simulink model "abc"  (R2016a)
settings: Solver=VariableStepAuto  StartTime=0.0  StopTime=end_time  RelTol=1e-3
values from neighbouring files (symbols this model uses):
  Lambdad = 1e-5    (= 1e-05)    [myModel_param.m]
  Lambdaq = 1e-5    (= 1e-05)    [myModel_param.m]
  Li = 0.16e-3    (= 0.00016)    [Model.m]    (also in myModel_param.m)
  ri = 0.1    [Model.m]    (also in myModel_param.m)
  s_1 = [0;0;0]    [myModel_param.m]
  s_2 = [1;0;0]    [myModel_param.m]
  s_3 = [1;1;0]    [myModel_param.m]
  s_4 = [0;1;0]    [myModel_param.m]
  s_5 = [0;1;1]    [myModel_param.m]
  s_6 = [0;0;1]    [myModel_param.m]
  s_7 = [1;0;1]    [myModel_param.m]
  s_8 = [1;1;1]    [myModel_param.m]
  Ts = 1e-4    (= 0.0001)    [Model.m]    (also in myModel_param.m = 0.001)
  wg = 61.25    [Model.m]    (also in myModel_param.m)
undefined symbols (not defined in the file or in its folder): Lambda1, Lambda2, LambdaP, P_ref
libraries: powerlib x12
settings Model: Creator=syf  LastModifiedBy=syf

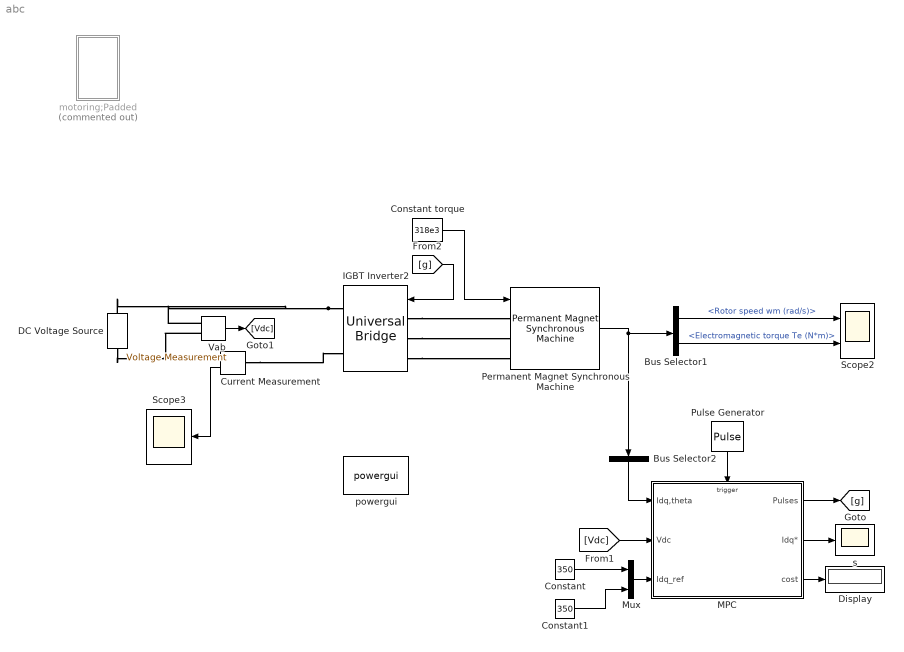
== system abc ==
  Bus Selector1 : BusSelector  OutputSignals=Rotor speed wm (rad/s),Electromagnetic torque Te (N*m)
  Bus Selector2 : BusSelector  OutputSignals=Stator current is_d (A),Stator current is_q (A),Rotor angle thetam (rad)  OutputAsBus=on
  Constant : Constant  Value=350
  Constant torque : Constant  Value=318e3
  Constant1 : Constant  Value=350
  Current Measurement : powerlib/Measurements/Current Measurement  PhasorSimulation=off  OutputType=Complex  PSBequivalent=0
  DC Voltage Source : powerlib/Electrical Sources/DC Voltage Source  Amplitude=540  Measurements=None
  Display : Display
  IGBT Inverter2 : powerlib/Power Electronics/Universal Bridge  Arms=3  SnubberResistance=1e6  SnubberCapacitance=1e-9  Device=IGBT / Diodes  Ron=1e-3  Lon=0  ForwardVoltages="[  0.8  0.8  ]"  ForwardVoltage=.8  GTOparameters=[ 1e-6 , 1e-6 ]  IGBTparameters=[ 1e-6 , 2e-6 ]  Measurements=All voltages and currents  Measurements_2=None  converterType=Rectifier
  MPC : Subsystem  TreatAsAtomicUnit=on
  Mux : Mux  Inputs=2
  Permanent Magnet Synchronous Machine : powerlib/Machines/Permanent Magnet Synchronous Machine  NbPhases=3  FluxDistribution=Sinusoidal  RotorType=Salient-pole  MechanicalLoad=Torque Tm  PresetModel=No  ShowDetailedParameters=on  MeasurementBus=off  Resistance=8.02e-3  Inductance=8.5e-3  dqInductances=[8.5e-3,8.5e-3]  La=2.07e-3  MachineConstant=Flux linkage established by magnets (V.s)  Flux=9.13  VoltageCst=43055.9693  TorqueCst=356.07  Flat=120  Mechanical=[1307e3 0.0004924 26 0]  PolePairs=4  InitialConditions=[0,0, 0,0]  InitialConditions5ph=[0 0 0 0 0 0]  TsPowergui=0  TsBlock=-1  RefAngle=Aligned with phase A axis (original Park)
  Pulse Generator : DiscretePulseGenerator  PulseType=Time based  Period=Ts*0.01  PulseWidth=20
  Scope2 : Scope  NumInputPorts=2
  Scope3 : Scope
  Vab : powerlib/Measurements/Voltage Measurement  Tag=PoWeRsYsTeMmEaSuReMeNt  PhasorSimulation=off  OutputType=Magnitude  PSBequivalent=0
  motoring;Padded : Subsystem  Commented=on
  powergui : powerlib/powergui  Priority=1  SimulationMode=Continuous  SolverType=Tustin/Backward Euler (TBE)  SampleTime=50e-6  frequency=60  SPID=on  DisableSnubberDevices=on  DisableRonSwitches=on  DisableVfSwitches=on  SwTol=0  DisplayEquations=off  Interpol=off  ExternalGateDelay=off  methode=off  Ts=10  FunctionMessages=off  echomessages=off  HookPort=off  EnableUseOfTLC=off  x0status=blocks  frequencyindice=0  Pbase=100e6  ErrMax=1e-4  Iterations=50  UnitsV=kV  UnitsW=MW  buscounter=0  RestoreLinks=warning  ResistiveCurrentMeasurement=off  Frange=[0:2:500]  Ylog=off  Xlog=on  ShowGrid=off  save=off  variable=ZData  structure=0  ZoomFFT=off  StartTime=0.0  cycles=1  DisplayStyle=1  fundamental=60  FreqAxis=off  MaxFrequency=1000  frequencyindicesteady=1  RmsSteady=1  display=off
  s : Scope
  wires:
  Bus Selector1/2 -> Scope2/2  "<Electromagnetic torque Te (N*m)>"
  Bus Selector1/1 -> Scope2/1  "<Rotor speed wm (rad/s)>"
  Pulse Generator/1 -> MPC/Trigger
  Permanent Magnet Synchronous Machine/1 -> Bus Selector2/1, Bus Selector1/1
  [Vdc] -> MPC/2(Vdc)
  MPC/1(Pulses) -> [g]
  Bus Selector2/1 -> MPC/1(Idq,theta)
  Constant torque/1 -> Permanent Magnet Synchronous Machine/1
  Vab/1 -> [Vdc]
  Current Measurement/1 -> Scope3/1
  MPC/2(Idq*) -> s/1
  MPC/3(cost) -> Display/1
  Mux/1 -> MPC/3(Idq_ref)
  Constant/1 -> Mux/1
  Constant1/1 -> Mux/2
  [g] -> IGBT Inverter2/1
  connections:
  Vab/LConn2 -- DC Voltage Source/LConn1 -- Current Measurement/RConn1
  IGBT Inverter2/RConn1 -- Vab/LConn1 -- DC Voltage Source/RConn1
  IGBT Inverter2/LConn3 -- Permanent Magnet Synchronous Machine/LConn3
  Current Measurement/LConn1 -- IGBT Inverter2/RConn2
  IGBT Inverter2/LConn2 -- Permanent Magnet Synchronous Machine/LConn2
  IGBT Inverter2/LConn1 -- Permanent Magnet Synchronous Machine/LConn1

== system abc/MPC ==
  Idq,theta : Inport
  Vdc : Inport  Port=2
  Idq_ref : Inport  Port=3
  Trigger : TriggerPort  VariantControl=Variant
  For Loop : Subsystem  TreatAsAtomicUnit=on
  Gate Pulse Translation for min sw : Subsystem
  Pulses : Outport
  Idq* : Outport  Port=2
  cost : Outport  Port=3
  wires:
  Idq,theta/1 -> For Loop/1(Idq,theta)
  Vdc/1 -> For Loop/2(Vdc)
  Gate Pulse Translation for min sw/1(pulses) -> Pulses/1
  For Loop/1(opti) -> Gate Pulse Translation for min sw/1(i)
  Idq_ref/1 -> For Loop/3(Idq_ref)
  For Loop/2(Idq*) -> Idq*/1
  For Loop/3(cost) -> cost/1

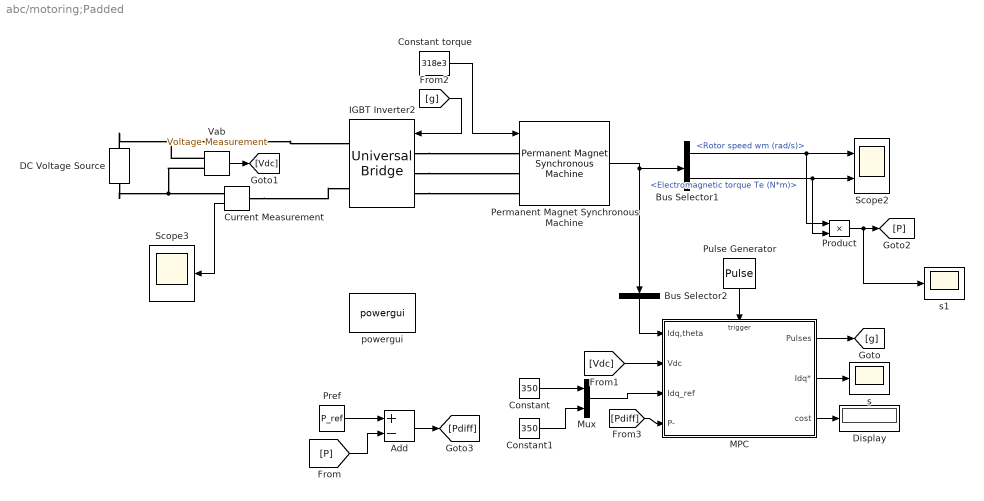
== system abc/motoring;Padded ==
  Add : Sum  Inputs=+-
  Bus Selector1 : BusSelector  OutputSignals=Rotor speed wm (rad/s),Electromagnetic torque Te (N*m)
  Bus Selector2 : BusSelector  OutputSignals=Stator current is_d (A),Stator current is_q (A),Rotor angle thetam (rad)  OutputAsBus=on
  Constant : Constant  Value=350
  Constant torque : Constant  Value=318e3
  Constant1 : Constant  Value=350
  Current Measurement : powerlib/Measurements/Current Measurement  PhasorSimulation=off  OutputType=Complex  PSBequivalent=0
  DC Voltage Source : powerlib/Electrical Sources/DC Voltage Source  Amplitude=540  Measurements=None
  Display : Display
  IGBT Inverter2 : powerlib/Power Electronics/Universal Bridge  Arms=3  SnubberResistance=1e6  SnubberCapacitance=1e-9  Device=IGBT / Diodes  Ron=1e-3  Lon=0  ForwardVoltages="[  0.8  0.8  ]"  ForwardVoltage=.8  GTOparameters=[ 1e-6 , 1e-6 ]  IGBTparameters=[ 1e-6 , 2e-6 ]  Measurements=All voltages and currents  Measurements_2=None  converterType=Rectifier
  MPC : Subsystem  TreatAsAtomicUnit=on
  Mux : Mux  Inputs=2
  Permanent Magnet Synchronous Machine : powerlib/Machines/Permanent Magnet Synchronous Machine  NbPhases=3  FluxDistribution=Sinusoidal  RotorType=Salient-pole  MechanicalLoad=Torque Tm  PresetModel=No  ShowDetailedParameters=on  MeasurementBus=off  Resistance=8.02e-3  Inductance=8.5e-3  dqInductances=[8.5e-3,8.5e-3]  La=2.07e-3  MachineConstant=Flux linkage established by magnets (V.s)  Flux=9.13  VoltageCst=43055.9693  TorqueCst=356.07  Flat=120  Mechanical=[1307e3 0.0004924 26 0]  PolePairs=4  InitialConditions=[0,0, 0,0]  InitialConditions5ph=[0 0 0 0 0 0]  TsPowergui=0  TsBlock=-1  RefAngle=Aligned with phase A axis (original Park)
  Pref : Constant  Value=P_ref
  Product : Product
  Pulse Generator : DiscretePulseGenerator  PulseType=Time based  Period=Ts*0.01  PulseWidth=20
  Scope2 : Scope  NumInputPorts=2
  Scope3 : Scope
  Vab : powerlib/Measurements/Voltage Measurement  Tag=PoWeRsYsTeMmEaSuReMeNt  PhasorSimulation=off  OutputType=Magnitude  PSBequivalent=0
  powergui : powerlib/powergui  Priority=1  SimulationMode=Continuous  SolverType=Tustin/Backward Euler (TBE)  SampleTime=50e-6  frequency=60  SPID=on  DisableSnubberDevices=on  DisableRonSwitches=on  DisableVfSwitches=on  SwTol=0  DisplayEquations=off  Interpol=off  ExternalGateDelay=off  methode=off  Ts=10  FunctionMessages=off  echomessages=off  HookPort=off  EnableUseOfTLC=off  x0status=blocks  frequencyindice=0  Pbase=100e6  ErrMax=1e-4  Iterations=50  UnitsV=kV  UnitsW=MW  buscounter=0  RestoreLinks=warning  ResistiveCurrentMeasurement=off  Frange=[0:2:500]  Ylog=off  Xlog=on  ShowGrid=off  save=off  variable=ZData  structure=0  ZoomFFT=off  StartTime=0.0  cycles=1  DisplayStyle=1  fundamental=60  FreqAxis=off  MaxFrequency=1000  frequencyindicesteady=1  RmsSteady=1  display=off
  s : Scope
  s1 : Scope
  wires:
  [g] -> IGBT Inverter2/1
  Constant1/1 -> Mux/2
  Constant/1 -> Mux/1
  Mux/1 -> MPC/3(Idq_ref)
  MPC/3(cost) -> Display/1
  MPC/2(Idq*) -> s/1
  Current Measurement/1 -> Scope3/1
  Vab/1 -> [Vdc]
  Constant torque/1 -> Permanent Magnet Synchronous Machine/1
  Bus Selector2/1 -> MPC/1(Idq,theta)
  MPC/1(Pulses) -> [g]
  [Vdc] -> MPC/2(Vdc)
  Permanent Magnet Synchronous Machine/1 -> Bus Selector1/1, Bus Selector2/1
  Pulse Generator/1 -> MPC/Trigger
  Bus Selector1/1 -> Product/1, Scope2/1  "<Rotor speed wm (rad/s)>"
  Bus Selector1/2 -> Product/2, Scope2/2  "<Electromagnetic torque Te (N*m)>"
  Product/1 -> s1/1, [P]
  Pref/1 -> Add/1
  [P] -> Add/2
  Add/1 -> [Pdiff]
  [Pdiff] -> MPC/4(P-)
  connections:
  IGBT Inverter2/LConn2 -- Permanent Magnet Synchronous Machine/LConn2
  Current Measurement/LConn1 -- IGBT Inverter2/RConn2
  DC Voltage Source/RConn1 -- IGBT Inverter2/RConn1 -- Vab/LConn1
  DC Voltage Source/LConn1 -- Vab/LConn2 -- Current Measurement/RConn1
  IGBT Inverter2/LConn1 -- Permanent Magnet Synchronous Machine/LConn1
  IGBT Inverter2/LConn3 -- Permanent Magnet Synchronous Machine/LConn3

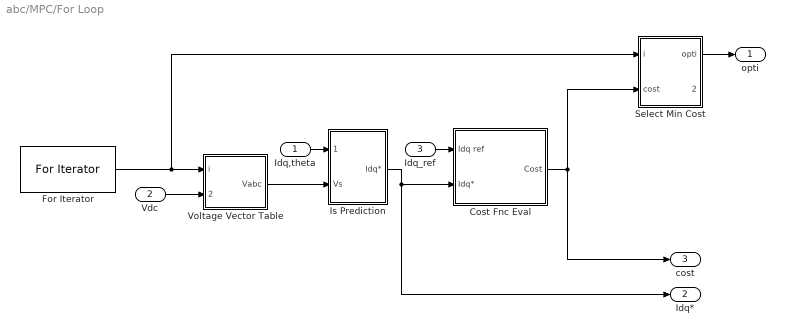
== system abc/MPC/For Loop ==
  Idq,theta : Inport
  Vdc : Inport  Port=2
  Idq_ref : Inport  Port=3
  Cost Fnc Eval : Subsystem
  For Iterator : ForIterator  IterationLimit=8  IterationVariableDataType=double
  Is Prediction : Subsystem
  Select Min Cost : Subsystem
  Voltage Vector Table : Subsystem
  opti : Outport
  Idq* : Outport  Port=2
  cost : Outport  Port=3
  wires:
  Select Min Cost/1(opti) -> opti/1
  Is Prediction/1(Idq*) -> Cost Fnc Eval/2("Idq* "), Idq*/1
  Idq,theta/1 -> Is Prediction/1(Idq,theta)
  Vdc/1 -> Voltage Vector Table/2(DC Link)
  Cost Fnc Eval/1(Cost) -> Select Min Cost/2(cost), cost/1
  For Iterator/1 -> Select Min Cost/1(i), Voltage Vector Table/1(i)
  Idq_ref/1 -> Cost Fnc Eval/1(Idq ref)
  Voltage Vector Table/1(Vabc) -> Is Prediction/2(Vs)

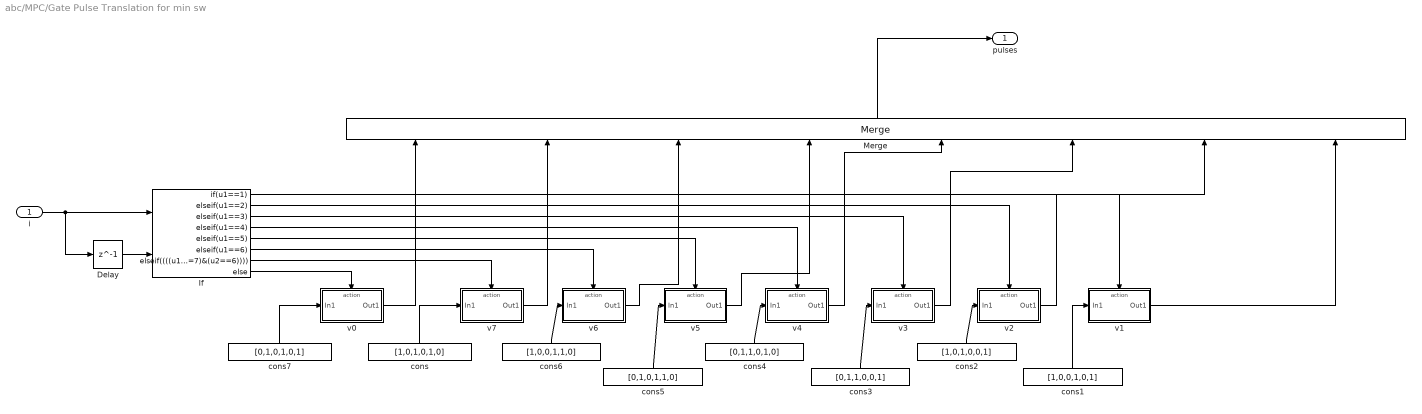
== system abc/MPC/Gate Pulse Translation for min sw ==
  i : Inport
  Delay : Delay  DelayLength=1  InitialCondition=0
  If : If  NumInputs=2  IfExpression=u1==1  ElseIfExpressions=u1==2, u1==3, u1==4, u1==5, u1==6,(((u1==7)&(u2==2)) | ((u1==7)&(u2==4)) | ((u1==7)&(u2==6)))
  Merge : Merge  Inputs=8
  cons : Constant  Value=[1,0,1,0,1,0]
  cons1 : Constant  Value=[1,0,0,1,0,1]
  cons2 : Constant  Value=[1,0,1,0,0,1]
  cons3 : Constant  Value=[0,1,1,0,0,1]
  cons4 : Constant  Value=[0,1,1,0,1,0]
  cons5 : Constant  Value=[0,1,0,1,1,0]
  cons6 : Constant  Value=[1,0,0,1,1,0]
  cons7 : Constant  Value=[0,1,0,1,0,1]
  v0 : Subsystem  TreatAsAtomicUnit=on
  v1 : Subsystem  TreatAsAtomicUnit=on
  v2 : Subsystem  TreatAsAtomicUnit=on
  v3 : Subsystem  TreatAsAtomicUnit=on
  v4 : Subsystem  TreatAsAtomicUnit=on
  v5 : Subsystem  TreatAsAtomicUnit=on
  v6 : Subsystem  TreatAsAtomicUnit=on
  v7 : Subsystem  TreatAsAtomicUnit=on
  pulses : Outport
  wires:
  i/1 -> Delay/1, If/1
  If/1 -> v1/Action
  Merge/1 -> pulses/1
  cons/1 -> v7/1(In1)
  If/3 -> v3/Action
  If/2 -> v2/Action
  If/4 -> v4/Action
  If/5 -> v5/Action
  If/7 -> v7/Action
  If/6 -> v6/Action
  cons1/1 -> v1/1(In1)
  cons2/1 -> v2/1(In1)
  cons3/1 -> v3/1(In1)
  cons4/1 -> v4/1(In1)
  cons5/1 -> v5/1(In1)
  cons6/1 -> v6/1(In1)
  Delay/1 -> If/2
  cons7/1 -> v0/1(In1)
  If/8 -> v0/Action
  v0/1(Out1) -> Merge/1
  v7/1(Out1) -> Merge/2
  v6/1(Out1) -> Merge/3
  v5/1(Out1) -> Merge/4
  v4/1(Out1) -> Merge/5
  v3/1(Out1) -> Merge/6
  v2/1(Out1) -> Merge/7
  v1/1(Out1) -> Merge/8

== system abc/motoring;Padded/MPC ==
  Idq,theta : Inport
  Vdc : Inport  Port=2
  Idq_ref : Inport  Port=3
  P- : Inport  Port=4
  Trigger : TriggerPort  VariantControl=Variant
  For Loop : Subsystem  TreatAsAtomicUnit=on
  Gate Pulse Translation for min sw : Subsystem
  Pulses : Outport
  Idq* : Outport  Port=2
  cost : Outport  Port=3
  wires:
  For Loop/3(cost) -> cost/1
  For Loop/2(Idq*) -> Idq*/1
  Idq_ref/1 -> For Loop/3(Idq_ref)
  For Loop/1(opti) -> Gate Pulse Translation for min sw/1(i)
  Gate Pulse Translation for min sw/1(pulses) -> Pulses/1
  Vdc/1 -> For Loop/2(Vdc)
  Idq,theta/1 -> For Loop/1(Idq,theta)
  P-/1 -> ?

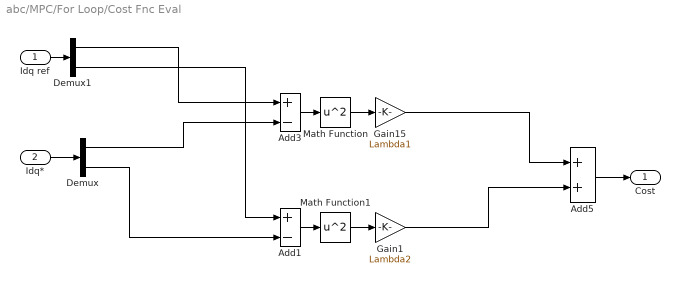
== system abc/MPC/For Loop/Cost Fnc Eval ==
  Idq ref : Inport
  "Idq* " : Inport  Port=2
  Add1 : Sum  Inputs=+-
  Add3 : Sum  Inputs=+-
  Add5 : Sum
  Demux : Demux  Outputs=2
  Demux1 : Demux  Outputs=2
  Gain1 : Gain  Gain=Lambda2
  Gain15 : Gain  Gain=Lambda1
  Math Function : Math  Operator=square  SaturateOnIntegerOverflow=on
  Math Function1 : Math  Operator=square  SaturateOnIntegerOverflow=on
  Cost : Outport
  wires:
  Demux1/1 -> Add3/1
  Gain1/1 -> Add5/2
  Add5/1 -> Cost/1
  Gain15/1 -> Add5/1
  Add1/1 -> Math Function1/1
  Demux1/2 -> Add1/1
  "Idq* "/1 -> Demux/1
  Demux/2 -> Add1/2
  Demux/1 -> Add3/2
  Add3/1 -> Math Function/1
  Math Function/1 -> Gain15/1
  Math Function1/1 -> Gain1/1
  Idq ref/1 -> Demux1/1

== system abc/MPC/For Loop/Is Prediction ==
  Idq,theta : Inport
  Vs : Inport  Port=2
  Demux : Demux  Outputs=2
  Demux1 : Demux  Outputs=2
  Id_pred : Subsystem
  Iq_pred : Subsystem
  MATLAB Function : MATLAB Function  TreatAsAtomicUnit=on
  Mux : Mux  Inputs=2
  Idq* : Outport
  wires:
  Demux1/1 -> Id_pred/2(Vd)
  Demux1/2 -> Iq_pred/2("Vq ")
  Id_pred/1(Id*) -> Mux/1
  Iq_pred/1(Iq*) -> Mux/2
  Mux/1 -> Idq*/1
  Idq,theta/1 -> Demux/1
  Demux/1 -> Iq_pred/1(Idq), Id_pred/1(Idq)
  Demux/2 -> MATLAB Function/1(theta)
  Vs/1 -> MATLAB Function/2(Vs)
  MATLAB Function/1(Vdq) -> Demux1/1

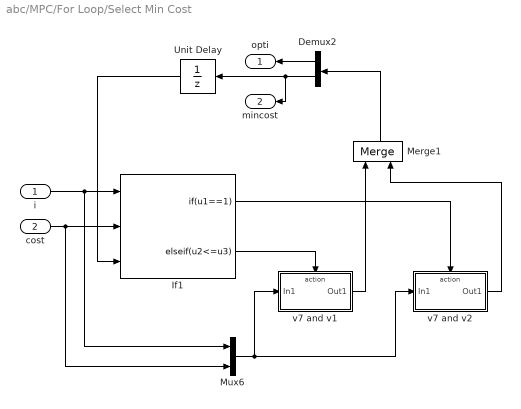
== system abc/MPC/For Loop/Select Min Cost ==
  i : Inport
  cost : Inport  Port=2
  Demux2 : Demux  Outputs=2
  If1 : If  NumInputs=3  IfExpression=u1==1  ElseIfExpressions=u2<=u3  ShowElse=off
  Merge1 : Merge
  Mux6 : Mux  Inputs=2
  Unit Delay : UnitDelay  SampleTime=-1
  v7 and v1 : Subsystem  TreatAsAtomicUnit=on
  v7 and v2 : Subsystem  TreatAsAtomicUnit=on
  opti : Outport
  mincost : Outport  Port=2
  wires:
  cost/1 -> Mux6/2, If1/2
  If1/1 -> v7 and v2/Action
  Unit Delay/1 -> If1/3
  i/1 -> Mux6/1, If1/1
  Mux6/1 -> v7 and v1/1(In1), v7 and v2/1(In1)
  Merge1/1 -> Demux2/1
  Demux2/2 -> mincost/1, Unit Delay/1
  If1/2 -> v7 and v1/Action
  v7 and v1/1(Out1) -> Merge1/1
  v7 and v2/1(Out1) -> Merge1/2
  Demux2/1 -> opti/1

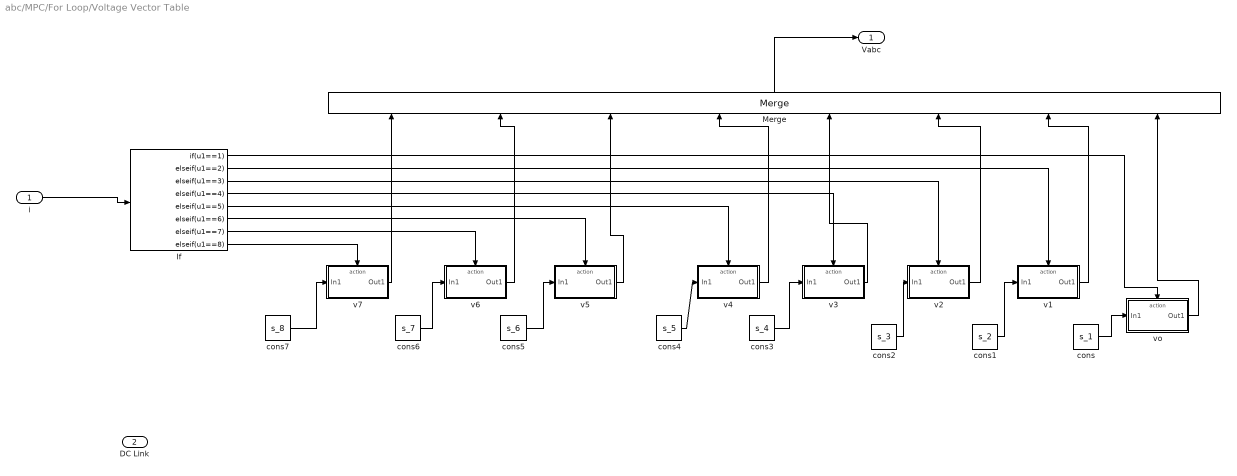
== system abc/MPC/For Loop/Voltage Vector Table ==
  i : Inport
  DC Link : Inport  Port=2
  If : If  IfExpression=u1==1  ElseIfExpressions=u1==2, u1==3, u1==4, u1==5, u1==6, u1==7,u1==8  ShowElse=off
  Merge : Merge  Inputs=8
  cons : Constant  Value=s_1
  cons1 : Constant  Value=s_2
  cons2 : Constant  Value=s_3
  cons3 : Constant  Value=s_4
  cons4 : Constant  Value=s_5
  cons5 : Constant  Value=s_6
  cons6 : Constant  Value=s_7
  cons7 : Constant  Value=s_8
  v1 : Subsystem  TreatAsAtomicUnit=on
  v2 : Subsystem  TreatAsAtomicUnit=on
  v3 : Subsystem  TreatAsAtomicUnit=on
  v4 : Subsystem  TreatAsAtomicUnit=on
  v5 : Subsystem  TreatAsAtomicUnit=on
  v6 : Subsystem  TreatAsAtomicUnit=on
  "v7 " : Subsystem  TreatAsAtomicUnit=on
  vo : Subsystem  TreatAsAtomicUnit=on
  Vabc : Outport
  wires:
  i/1 -> If/1
  cons7/1 -> "v7 "/1(In1)
  v1/1(Out1) -> Merge/7
  v2/1(Out1) -> Merge/6
  v3/1(Out1) -> Merge/5
  v4/1(Out1) -> Merge/4
  v5/1(Out1) -> Merge/3
  v6/1(Out1) -> Merge/2
  "v7 "/1(Out1) -> Merge/1
  Merge/1 -> Vabc/1
  cons/1 -> vo/1(In1)
  vo/1(Out1) -> Merge/8
  cons6/1 -> v6/1(In1)
  cons5/1 -> v5/1(In1)
  cons4/1 -> v4/1(In1)
  cons3/1 -> v3/1(In1)
  cons2/1 -> v2/1(In1)
  cons1/1 -> v1/1(In1)
  If/8 -> "v7 "/Action
  If/7 -> v6/Action
  If/6 -> v5/Action
  If/5 -> v4/Action
  If/4 -> v3/Action
  If/3 -> v2/Action
  If/2 -> v1/Action
  If/1 -> vo/Action

== system abc/MPC/Gate Pulse Translation for min sw/v0 ==
  In1 : Inport
  Action Port : ActionPort  ActionType=else
  Out1 : Outport
  wires:
  In1/1 -> Out1/1

== system abc/MPC/Gate Pulse Translation for min sw/v1 ==
  In1 : Inport
  Action Port : ActionPort  ActionType=then
  Out1 : Outport
  wires:
  In1/1 -> Out1/1

== system abc/MPC/Gate Pulse Translation for min sw/v2 ==
  In1 : Inport
  Action Port : ActionPort  ActionType=elseif
  Out1 : Outport
  wires:
  In1/1 -> Out1/1

== system abc/MPC/Gate Pulse Translation for min sw/v3 ==
  In1 : Inport
  Action Port : ActionPort  ActionType=elseif
  Out1 : Outport
  wires:
  In1/1 -> Out1/1

== system abc/MPC/Gate Pulse Translation for min sw/v4 ==
  In1 : Inport
  Action Port : ActionPort  ActionType=elseif
  Out1 : Outport
  wires:
  In1/1 -> Out1/1

== system abc/MPC/Gate Pulse Translation for min sw/v5 ==
  In1 : Inport
  Action Port : ActionPort  ActionType=elseif
  Out1 : Outport
  wires:
  In1/1 -> Out1/1

== system abc/MPC/Gate Pulse Translation for min sw/v6 ==
  In1 : Inport
  Action Port : ActionPort  ActionType=elseif
  Out1 : Outport
  wires:
  In1/1 -> Out1/1

== system abc/MPC/Gate Pulse Translation for min sw/v7 ==
  In1 : Inport
  Action Port : ActionPort  ActionType=elseif
  Out1 : Outport
  wires:
  In1/1 -> Out1/1

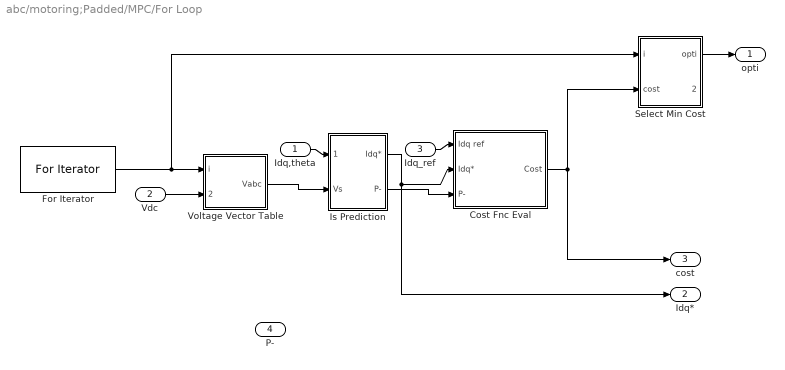
== system abc/motoring;Padded/MPC/For Loop ==
  Idq,theta : Inport
  Vdc : Inport  Port=2
  Idq_ref : Inport  Port=3
  P- : Inport  Port=4
  Cost Fnc Eval : Subsystem
  For Iterator : ForIterator  IterationLimit=8  IterationVariableDataType=double
  Is Prediction : Subsystem
  Select Min Cost : Subsystem
  Voltage Vector Table : Subsystem
  opti : Outport
  Idq* : Outport  Port=2
  cost : Outport  Port=3
  wires:
  Voltage Vector Table/1(Vabc) -> Is Prediction/2(Vs)
  Idq_ref/1 -> Cost Fnc Eval/1(Idq ref)
  For Iterator/1 -> Voltage Vector Table/1(i), Select Min Cost/1(i)
  Cost Fnc Eval/1(Cost) -> cost/1, Select Min Cost/2(cost)
  Vdc/1 -> Voltage Vector Table/2(DC Link)
  Idq,theta/1 -> Is Prediction/1(Idq,theta)
  Is Prediction/1(Idq*) -> Idq*/1, Cost Fnc Eval/2("Idq* ")
  Select Min Cost/1(opti) -> opti/1
  Is Prediction/2(P-) -> Cost Fnc Eval/3(P-)

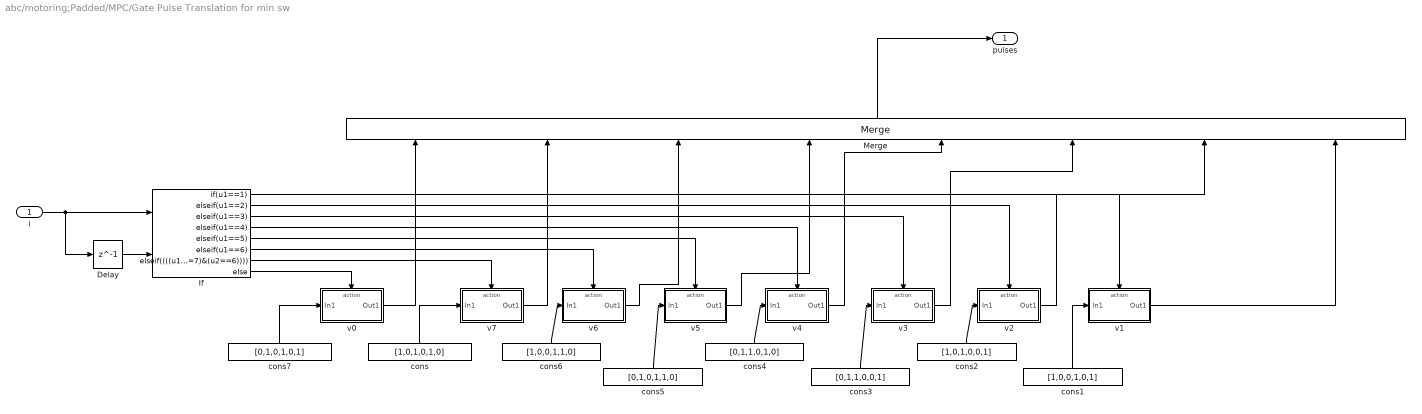
== system abc/motoring;Padded/MPC/Gate Pulse Translation for min sw ==
  i : Inport
  Delay : Delay  DelayLength=1  InitialCondition=0
  If : If  NumInputs=2  IfExpression=u1==1  ElseIfExpressions=u1==2, u1==3, u1==4, u1==5, u1==6,(((u1==7)&(u2==2)) | ((u1==7)&(u2==4)) | ((u1==7)&(u2==6)))
  Merge : Merge  Inputs=8
  cons : Constant  Value=[1,0,1,0,1,0]
  cons1 : Constant  Value=[1,0,0,1,0,1]
  cons2 : Constant  Value=[1,0,1,0,0,1]
  cons3 : Constant  Value=[0,1,1,0,0,1]
  cons4 : Constant  Value=[0,1,1,0,1,0]
  cons5 : Constant  Value=[0,1,0,1,1,0]
  cons6 : Constant  Value=[1,0,0,1,1,0]
  cons7 : Constant  Value=[0,1,0,1,0,1]
  v0 : Subsystem  TreatAsAtomicUnit=on
  v1 : Subsystem  TreatAsAtomicUnit=on
  v2 : Subsystem  TreatAsAtomicUnit=on
  v3 : Subsystem  TreatAsAtomicUnit=on
  v4 : Subsystem  TreatAsAtomicUnit=on
  v5 : Subsystem  TreatAsAtomicUnit=on
  v6 : Subsystem  TreatAsAtomicUnit=on
  v7 : Subsystem  TreatAsAtomicUnit=on
  pulses : Outport
  wires:
  v1/1(Out1) -> Merge/8
  v2/1(Out1) -> Merge/7
  v3/1(Out1) -> Merge/6
  v4/1(Out1) -> Merge/5
  v5/1(Out1) -> Merge/4
  v6/1(Out1) -> Merge/3
  v7/1(Out1) -> Merge/2
  v0/1(Out1) -> Merge/1
  If/8 -> v0/Action
  cons7/1 -> v0/1(In1)
  Delay/1 -> If/2
  cons6/1 -> v6/1(In1)
  cons5/1 -> v5/1(In1)
  cons4/1 -> v4/1(In1)
  cons3/1 -> v3/1(In1)
  cons2/1 -> v2/1(In1)
  cons1/1 -> v1/1(In1)
  If/6 -> v6/Action
  If/7 -> v7/Action
  If/5 -> v5/Action
  If/4 -> v4/Action
  If/2 -> v2/Action
  If/3 -> v3/Action
  cons/1 -> v7/1(In1)
  Merge/1 -> pulses/1
  If/1 -> v1/Action
  i/1 -> If/1, Delay/1

== system abc/MPC/For Loop/Is Prediction/Id_pred ==
  Idq : Inport
  Vd : Inport  Port=2
  Add : Sum  Inputs=+++
  Demux : Demux  Outputs=2
  Gain : Gain  Gain=1-ri*Ts/Li
  Gain1 : Gain  Gain=wg*Ts
  Gain2 : Gain  Gain=Ts/Li
  Id* : Outport
  wires:
  Idq/1 -> Demux/1
  Demux/1 -> Gain/1
  Demux/2 -> Gain1/1
  Vd/1 -> Gain2/1
  Gain/1 -> Add/1
  Gain1/1 -> Add/2
  Gain2/1 -> Add/3
  Add/1 -> Id*/1

== system abc/MPC/For Loop/Is Prediction/Iq_pred ==
  Idq : Inport
  "Vq " : Inport  Port=2
  Add : Sum  Inputs=+++
  Demux : Demux  Outputs=2
  Gain : Gain  Gain=-wg*Ts
  Gain1 : Gain  Gain=1-ri*Ts/Li
  Gain2 : Gain  Gain=Ts/Li
  Iq* : Outport
  wires:
  Add/1 -> Iq*/1
  Gain2/1 -> Add/3
  Gain1/1 -> Add/2
  Gain/1 -> Add/1
  "Vq "/1 -> Gain2/1
  Demux/2 -> Gain1/1
  Demux/1 -> Gain/1
  Idq/1 -> Demux/1

== system abc/MPC/For Loop/Select Min Cost/v7 and v1 ==
  In1 : Inport
  Action Port : ActionPort  ActionType=elseif
  Out1 : Outport
  wires:
  In1/1 -> Out1/1

== system abc/MPC/For Loop/Select Min Cost/v7 and v2 ==
  In1 : Inport
  Action Port : ActionPort  ActionType=then
  Out1 : Outport
  wires:
  In1/1 -> Out1/1

== system abc/MPC/For Loop/Voltage Vector Table/v1 ==
  In1 : Inport
  Action Port : ActionPort  ActionType=elseif
  Out1 : Outport
  wires:
  In1/1 -> Out1/1

== system abc/MPC/For Loop/Voltage Vector Table/v2 ==
  In1 : Inport
  Action Port : ActionPort  ActionType=elseif
  Out1 : Outport
  wires:
  In1/1 -> Out1/1

== system abc/MPC/For Loop/Voltage Vector Table/v3 ==
  In1 : Inport
  Action Port : ActionPort  ActionType=elseif
  Out1 : Outport
  wires:
  In1/1 -> Out1/1

== system abc/MPC/For Loop/Voltage Vector Table/v4 ==
  In1 : Inport
  Action Port : ActionPort  ActionType=elseif
  Out1 : Outport
  wires:
  In1/1 -> Out1/1

== system abc/MPC/For Loop/Voltage Vector Table/v5 ==
  In1 : Inport
  Action Port : ActionPort  ActionType=elseif
  Out1 : Outport
  wires:
  In1/1 -> Out1/1

== system abc/MPC/For Loop/Voltage Vector Table/v6 ==
  In1 : Inport
  Action Port : ActionPort  ActionType=elseif
  Out1 : Outport
  wires:
  In1/1 -> Out1/1

== system abc/MPC/For Loop/Voltage Vector Table/v7  ==
  In1 : Inport
  Action Port : ActionPort  ActionType=elseif
  Out1 : Outport
  wires:
  In1/1 -> Out1/1

== system abc/MPC/For Loop/Voltage Vector Table/vo ==
  In1 : Inport
  Action Port : ActionPort  ActionType=then
  Out1 : Outport
  wires:
  In1/1 -> Out1/1

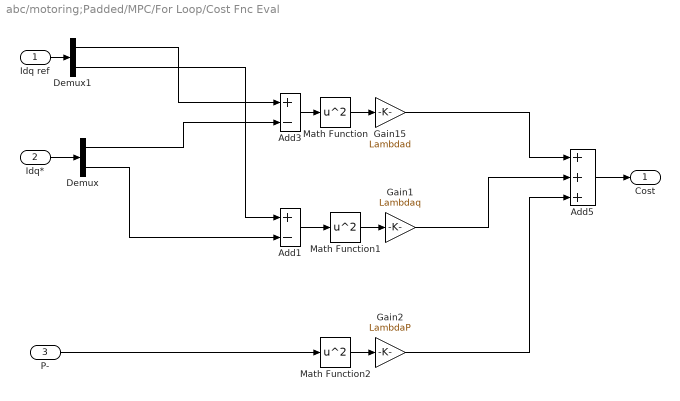
== system abc/motoring;Padded/MPC/For Loop/Cost Fnc Eval ==
  Idq ref : Inport
  "Idq* " : Inport  Port=2
  P- : Inport  Port=3
  Add1 : Sum  Inputs=+-
  Add3 : Sum  Inputs=+-
  Add5 : Sum  Inputs=+++
  Demux : Demux  Outputs=2
  Demux1 : Demux  Outputs=2
  Gain1 : Gain  Gain=Lambdaq
  Gain15 : Gain  Gain=Lambdad
  Gain2 : Gain  Gain=LambdaP
  Math Function : Math  Operator=square  SaturateOnIntegerOverflow=on
  Math Function1 : Math  Operator=square  SaturateOnIntegerOverflow=on
  Math Function2 : Math  Operator=square  SaturateOnIntegerOverflow=on
  Cost : Outport
  wires:
  Idq ref/1 -> Demux1/1
  Math Function1/1 -> Gain1/1
  Math Function/1 -> Gain15/1
  Add3/1 -> Math Function/1
  Demux/1 -> Add3/2
  Demux/2 -> Add1/2
  "Idq* "/1 -> Demux/1
  Demux1/2 -> Add1/1
  Add1/1 -> Math Function1/1
  Gain15/1 -> Add5/1
  Add5/1 -> Cost/1
  Gain1/1 -> Add5/2
  Demux1/1 -> Add3/1
  Math Function2/1 -> Gain2/1
  P-/1 -> Math Function2/1
  Gain2/1 -> Add5/3

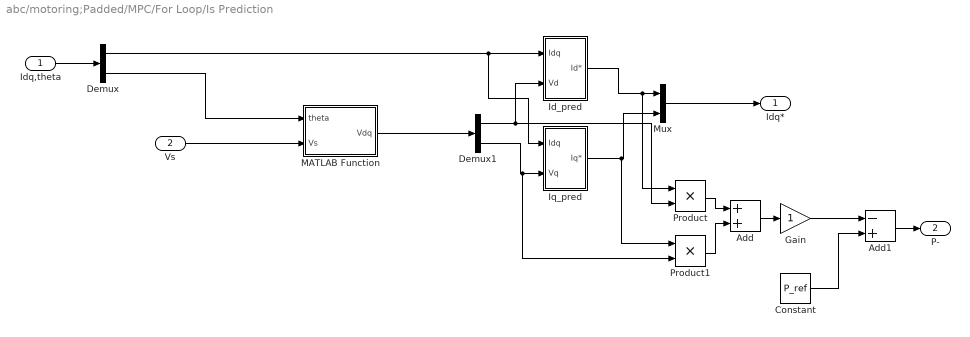
== system abc/motoring;Padded/MPC/For Loop/Is Prediction ==
  Idq,theta : Inport
  Vs : Inport  Port=2
  Add : Sum
  Add1 : Sum  Inputs=-+
  Constant : Constant  Value=P_ref
  Demux : Demux  Outputs=2
  Demux1 : Demux  Outputs=2
  Gain : Gain
  Id_pred : Subsystem
  Iq_pred : Subsystem
  MATLAB Function : MATLAB Function  TreatAsAtomicUnit=on
  Mux : Mux  Inputs=2
  Product : Product
  Product1 : Product
  Idq* : Outport
  P- : Outport  Port=2
  wires:
  MATLAB Function/1(Vdq) -> Demux1/1
  Vs/1 -> MATLAB Function/2(Vs)
  Demux/2 -> MATLAB Function/1(theta)
  Demux/1 -> Id_pred/1(Idq), Iq_pred/1(Idq)
  Idq,theta/1 -> Demux/1
  Mux/1 -> Idq*/1
  Iq_pred/1(Iq*) -> Product1/1, Mux/2
  Id_pred/1(Id*) -> Product/1, Mux/1
  Demux1/2 -> Product1/2, Iq_pred/2("Vq ")
  Demux1/1 -> Product/2, Id_pred/2(Vd)
  Product/1 -> Add/1
  Product1/1 -> Add/2
  Add/1 -> Gain/1
  Gain/1 -> Add1/1
  Constant/1 -> Add1/2
  Add1/1 -> P-/1

== system abc/motoring;Padded/MPC/For Loop/Select Min Cost ==
  i : Inport
  cost : Inport  Port=2
  Demux2 : Demux  Outputs=2
  If1 : If  NumInputs=3  IfExpression=u1==1  ElseIfExpressions=u2<=u3  ShowElse=off
  Merge1 : Merge
  Mux6 : Mux  Inputs=2
  Unit Delay : UnitDelay  SampleTime=-1
  v7 and v1 : Subsystem  TreatAsAtomicUnit=on
  v7 and v2 : Subsystem  TreatAsAtomicUnit=on
  opti : Outport
  mincost : Outport  Port=2
  wires:
  Demux2/1 -> opti/1
  v7 and v2/1(Out1) -> Merge1/2
  v7 and v1/1(Out1) -> Merge1/1
  If1/2 -> v7 and v1/Action
  Demux2/2 -> Unit Delay/1, mincost/1
  Merge1/1 -> Demux2/1
  Mux6/1 -> v7 and v2/1(In1), v7 and v1/1(In1)
  i/1 -> If1/1, Mux6/1
  Unit Delay/1 -> If1/3
  If1/1 -> v7 and v2/Action
  cost/1 -> If1/2, Mux6/2

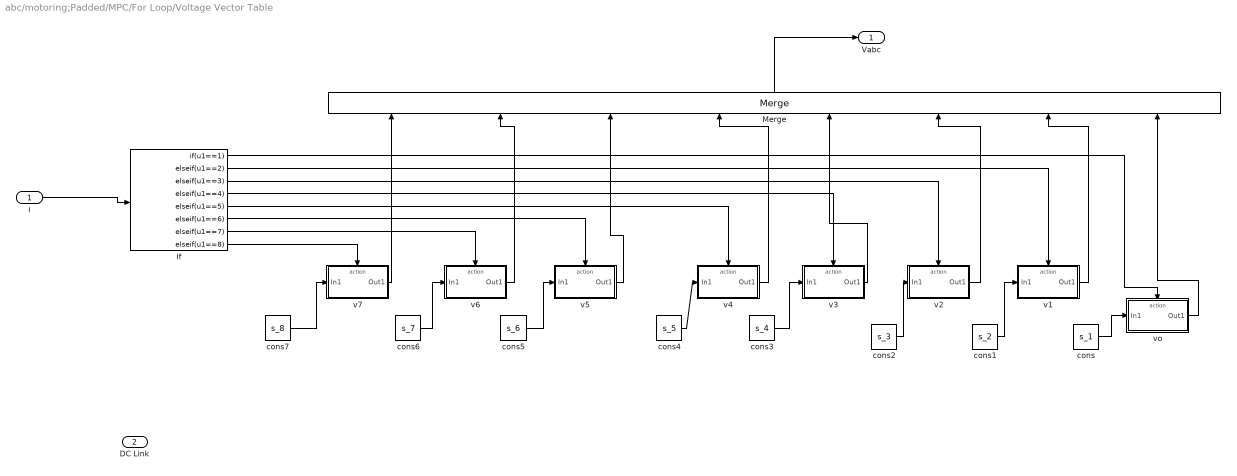
== system abc/motoring;Padded/MPC/For Loop/Voltage Vector Table ==
  i : Inport
  DC Link : Inport  Port=2
  If : If  IfExpression=u1==1  ElseIfExpressions=u1==2, u1==3, u1==4, u1==5, u1==6, u1==7,u1==8  ShowElse=off
  Merge : Merge  Inputs=8
  cons : Constant  Value=s_1
  cons1 : Constant  Value=s_2
  cons2 : Constant  Value=s_3
  cons3 : Constant  Value=s_4
  cons4 : Constant  Value=s_5
  cons5 : Constant  Value=s_6
  cons6 : Constant  Value=s_7
  cons7 : Constant  Value=s_8
  v1 : Subsystem  TreatAsAtomicUnit=on
  v2 : Subsystem  TreatAsAtomicUnit=on
  v3 : Subsystem  TreatAsAtomicUnit=on
  v4 : Subsystem  TreatAsAtomicUnit=on
  v5 : Subsystem  TreatAsAtomicUnit=on
  v6 : Subsystem  TreatAsAtomicUnit=on
  "v7 " : Subsystem  TreatAsAtomicUnit=on
  vo : Subsystem  TreatAsAtomicUnit=on
  Vabc : Outport
  wires:
  If/1 -> vo/Action
  If/2 -> v1/Action
  If/3 -> v2/Action
  If/4 -> v3/Action
  If/5 -> v4/Action
  If/6 -> v5/Action
  If/7 -> v6/Action
  If/8 -> "v7 "/Action
  cons1/1 -> v1/1(In1)
  cons2/1 -> v2/1(In1)
  cons3/1 -> v3/1(In1)
  cons4/1 -> v4/1(In1)
  cons5/1 -> v5/1(In1)
  cons6/1 -> v6/1(In1)
  vo/1(Out1) -> Merge/8
  cons/1 -> vo/1(In1)
  Merge/1 -> Vabc/1
  "v7 "/1(Out1) -> Merge/1
  v6/1(Out1) -> Merge/2
  v5/1(Out1) -> Merge/3
  v4/1(Out1) -> Merge/4
  v3/1(Out1) -> Merge/5
  v2/1(Out1) -> Merge/6
  v1/1(Out1) -> Merge/7
  cons7/1 -> "v7 "/1(In1)
  i/1 -> If/1

== system abc/motoring;Padded/MPC/Gate Pulse Translation for min sw/v0 ==
  In1 : Inport
  Action Port : ActionPort  ActionType=else
  Out1 : Outport
  wires:
  In1/1 -> Out1/1

== system abc/motoring;Padded/MPC/Gate Pulse Translation for min sw/v1 ==
  In1 : Inport
  Action Port : ActionPort  ActionType=then
  Out1 : Outport
  wires:
  In1/1 -> Out1/1

== system abc/motoring;Padded/MPC/Gate Pulse Translation for min sw/v2 ==
  In1 : Inport
  Action Port : ActionPort  ActionType=elseif
  Out1 : Outport
  wires:
  In1/1 -> Out1/1

== system abc/motoring;Padded/MPC/Gate Pulse Translation for min sw/v3 ==
  In1 : Inport
  Action Port : ActionPort  ActionType=elseif
  Out1 : Outport
  wires:
  In1/1 -> Out1/1

== system abc/motoring;Padded/MPC/Gate Pulse Translation for min sw/v4 ==
  In1 : Inport
  Action Port : ActionPort  ActionType=elseif
  Out1 : Outport
  wires:
  In1/1 -> Out1/1

== system abc/motoring;Padded/MPC/Gate Pulse Translation for min sw/v5 ==
  In1 : Inport
  Action Port : ActionPort  ActionType=elseif
  Out1 : Outport
  wires:
  In1/1 -> Out1/1

== system abc/motoring;Padded/MPC/Gate Pulse Translation for min sw/v6 ==
  In1 : Inport
  Action Port : ActionPort  ActionType=elseif
  Out1 : Outport
  wires:
  In1/1 -> Out1/1

== system abc/motoring;Padded/MPC/Gate Pulse Translation for min sw/v7 ==
  In1 : Inport
  Action Port : ActionPort  ActionType=elseif
  Out1 : Outport
  wires:
  In1/1 -> Out1/1

== system abc/motoring;Padded/MPC/For Loop/Is Prediction/Id_pred ==
  Idq : Inport
  Vd : Inport  Port=2
  Add : Sum  Inputs=+++
  Demux : Demux  Outputs=2
  Gain : Gain  Gain=1-ri*Ts/Li
  Gain1 : Gain  Gain=wg*Ts
  Gain2 : Gain  Gain=Ts/Li
  Id* : Outport
  wires:
  Add/1 -> Id*/1
  Gain2/1 -> Add/3
  Gain1/1 -> Add/2
  Gain/1 -> Add/1
  Vd/1 -> Gain2/1
  Demux/2 -> Gain1/1
  Demux/1 -> Gain/1
  Idq/1 -> Demux/1

== system abc/motoring;Padded/MPC/For Loop/Is Prediction/Iq_pred ==
  Idq : Inport
  "Vq " : Inport  Port=2
  Add : Sum  Inputs=+++
  Demux : Demux  Outputs=2
  Gain : Gain  Gain=-wg*Ts
  Gain1 : Gain  Gain=1-ri*Ts/Li
  Gain2 : Gain  Gain=Ts/Li
  Iq* : Outport
  wires:
  Idq/1 -> Demux/1
  Demux/1 -> Gain/1
  Demux/2 -> Gain1/1
  "Vq "/1 -> Gain2/1
  Gain/1 -> Add/1
  Gain1/1 -> Add/2
  Gain2/1 -> Add/3
  Add/1 -> Iq*/1

== system abc/motoring;Padded/MPC/For Loop/Select Min Cost/v7 and v1 ==
  In1 : Inport
  Action Port : ActionPort  ActionType=elseif
  Out1 : Outport
  wires:
  In1/1 -> Out1/1

== system abc/motoring;Padded/MPC/For Loop/Select Min Cost/v7 and v2 ==
  In1 : Inport
  Action Port : ActionPort  ActionType=then
  Out1 : Outport
  wires:
  In1/1 -> Out1/1

== system abc/motoring;Padded/MPC/For Loop/Voltage Vector Table/v1 ==
  In1 : Inport
  Action Port : ActionPort  ActionType=elseif
  Out1 : Outport
  wires:
  In1/1 -> Out1/1

== system abc/motoring;Padded/MPC/For Loop/Voltage Vector Table/v2 ==
  In1 : Inport
  Action Port : ActionPort  ActionType=elseif
  Out1 : Outport
  wires:
  In1/1 -> Out1/1

== system abc/motoring;Padded/MPC/For Loop/Voltage Vector Table/v3 ==
  In1 : Inport
  Action Port : ActionPort  ActionType=elseif
  Out1 : Outport
  wires:
  In1/1 -> Out1/1

== system abc/motoring;Padded/MPC/For Loop/Voltage Vector Table/v4 ==
  In1 : Inport
  Action Port : ActionPort  ActionType=elseif
  Out1 : Outport
  wires:
  In1/1 -> Out1/1

== system abc/motoring;Padded/MPC/For Loop/Voltage Vector Table/v5 ==
  In1 : Inport
  Action Port : ActionPort  ActionType=elseif
  Out1 : Outport
  wires:
  In1/1 -> Out1/1

== system abc/motoring;Padded/MPC/For Loop/Voltage Vector Table/v6 ==
  In1 : Inport
  Action Port : ActionPort  ActionType=elseif
  Out1 : Outport
  wires:
  In1/1 -> Out1/1

== system abc/motoring;Padded/MPC/For Loop/Voltage Vector Table/v7  ==
  In1 : Inport
  Action Port : ActionPort  ActionType=elseif
  Out1 : Outport
  wires:
  In1/1 -> Out1/1

== system abc/motoring;Padded/MPC/For Loop/Voltage Vector Table/vo ==
  In1 : Inport
  Action Port : ActionPort  ActionType=then
  Out1 : Outport
  wires:
  In1/1 -> Out1/1

== matlab function abc/motoring;Padded/MPC/For Loop/Is Prediction/MATLAB Function ==
  data: theta input; Vdq output size=[2,1]; Vs input size=[3,1]
function Vdq = fcn(theta, Vs)
Talph=2/3*[1 -0.5 -0.5; 0 sqrt(3)/2 -sqrt(3)/2];
Tdq=[cos(theta) sin(theta); -sin(theta) cos(theta)];

Vdq = Tdq*Talph*Vs;

== matlab function abc/MPC/For Loop/Is Prediction/MATLAB Function ==
  data: theta input; Vdq output size=[2,1]; Vs input size=[3,1]
function Vdq = fcn(theta, Vs)
Talph=2/3*[1 -0.5 -0.5; 0 sqrt(3)/2 -sqrt(3)/2];
Tdq=[cos(theta) sin(theta); -sin(theta) cos(theta)];

Vdq = Tdq*Talph*Vs;
